simulink model "pll_8"  (Simulink 3.00)
settings: Solver=ode45  SolverMode=SingleTasking  StartTime=0.0  StopTime=10.0  RelTol=1e-3  AbsTol=1e-6

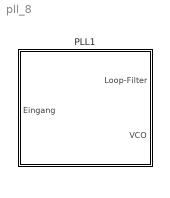
== system pll_8 ==
  PLL1 : Subsystem  mask(PLL-Schleife){f0=, ph_fehler=, kvco=, tau=}
      mask prompts: f0 "Ruhefrequenz"; ph_fehler "Phasenfehler-VCO"; kvco "Übertragungsfaktor-VCO"; tau "Zeitkonstante-Filter"
      mask help: Es wird eine analoge PLL-Schleife simuliert. Der Phasen-Detektor besteht aus einem Multiplizierer.
      mask init:
      | t = [0:0.1:2*pi,0];
      | x = cos(t);    y = sin(t);
      mask Help:
      | Pll-Schleife bestehend aus einem Multiplizierer als Phasen-Detektor, Tiefpaßfilter erster Ordnung und VCO. Die Parameter sind:
      | tau = Zeitkonstante des Filters
      | kvco = Übertragungsfaktor des VCOs
      | ph_fehler = Anfangsphasenfehler des VCO
      | f0 = Ruhefrequenz
      mask Display:
      | plot(0.25+0.1*x, 0.7+0.1*y);
      | plot([0.05,0.15], [0.7,0.7]);    plot([0.35,0.55],[0.7,0.7]);
      | plot([0.55,0.8,0.8,0.55,0.55],[0.6,0.6,0.8,0.8,0.6]);    plot([0.8,0.9,0.9,0.65],...
      | [0.7,0.7,0.350.35]);     plot([0.4,0.65,0.65,0.4,0.4],[0.25,0.25,0.45,0.45,0.25]);
      | plot([0.4,0.25,0.25],[0.35,0.35,0.6]);
      | text(0.23,0.70,'PD');    plot([0.15,0.1,0.1,0.15],[0.7, 0.725,0.675,0.7]);
      | text(0.6, 0.70,'TP');     plot([0.25,0.225,0.275,0.25],[0.6,0.55,0.55,0.6]);
      | text(0.45, 0.35,'VCO');
      | text(0.8, 0.2,'VCO');
      | text(0.60, 0.90,'Loop-Filter'); text(0.05, 0.45,'Eing.');

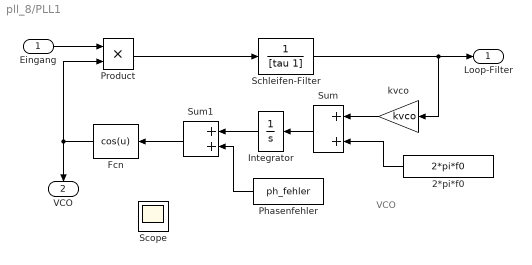
== system pll_8/PLL1 ==
  note: VCO
  Eingang : Inport  Port=1  PortWidth=-1  SampleTime=-1  DataType=auto
      settings: SignalType=auto
  2*pi*f0 : Constant  Orientation=left  Value=2*pi*f0
  Fcn : Fcn  Orientation=left  Expr=cos(u)
  Integrator : Integrator  Orientation=left  ExternalReset=none  InitialConditionSource=internal  InitialCondition=0  LimitOutput=off  UpperSaturationLimit=inf  LowerSaturationLimit=-inf  ShowSaturationPort=off  ShowStatePort=off  AbsoluteTolerance=auto
  Phasenfehler : Constant  Orientation=left  Value=ph_fehler
  Product : Product  Inputs=2  SaturateOnIntegerOverflow=on
  Schleifen-Filter : TransferFcn  Numerator=[1]  Denominator=[tau 1]
  Scope : Scope
      settings: Floating=on  TickLabels=on  TimeRange=0.1  YMin=-5  YMax=5  SaveToWorkspace=off  SaveName=ScopeData  DataFormat=Matrix
  Sum : Sum  Orientation=left  Inputs=++  SaturateOnIntegerOverflow=on
  Sum1 : Sum  Orientation=left  Inputs=++  SaturateOnIntegerOverflow=on
  kvco : Gain  Orientation=left  Gain=kvco  SaturateOnIntegerOverflow=on
  Loop-Filter : Outport  Port=1  InitialOutput=0
  " VCO" : Outport  Orientation=down  Port=2  InitialOutput=0
  wires:
  Integrator/1 -> Sum1/1
  Phasenfehler/1 -> Sum1/2
  Schleifen-Filter/1 -> Loop-Filter/1, kvco/1
  kvco/1 -> Sum/1
  2*pi*f0/1 -> Sum/2
  Sum/1 -> Integrator/1
  Product/1 -> Schleifen-Filter/1
  Sum1/1 -> Fcn/1
  Eingang/1 -> Product/1
  Fcn/1 -> " VCO"/1, Product/2
